simulink model "sim_demo"  (Simulink 8.2)
settings: Solver=ode45  StartTime=0.0  StopTime=10.0  RelTol=1e-3
libraries: simulink x1
settings Model: Creator=DR_C  LastModifiedBy=DR_C
settings DebuggingCC: FcnCallInpInsideContextMsg=EnableAllAsWarning
settings GRTTargetCC: CombineOutputUpdateFcns=on  GRTInterface=off

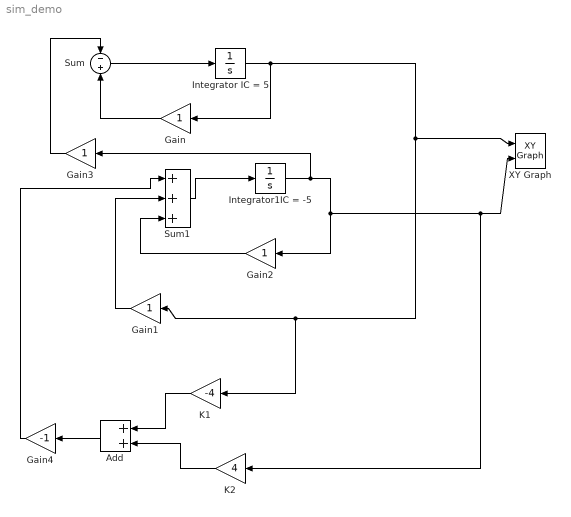
== system sim_demo ==
  Add : Sum
  Gain{,1..3} (4 alike) : Gain
  Gain4 : Gain  Gain=-1
  Integrator IC = 5 : Integrator  InitialCondition=5
  Integrator1IC = -5 : Integrator  InitialCondition=-5
  K1 : Gain  Gain=-4
  K2 : Gain  Gain=4
  Sum : Sum  Inputs=-+
  Sum1 : Sum  Inputs=+++
  XY Graph : simulink/Sinks/XY Graph  xmin=-10  xmax=10  ymin=-10  ymax=10  st=-1
  wires:
  Sum/1 -> Integrator IC = 5/1
  Gain/1 -> Sum/2
  Integrator IC = 5/1 -> Gain/1, XY Graph/1, Gain1/1, K1/1
  Sum1/1 -> Integrator1IC = -5/1
  Integrator1IC = -5/1 -> Gain3/1, Gain2/1, XY Graph/2, K2/1
  Gain3/1 -> Sum/1
  Gain2/1 -> Sum1/3
  Gain1/1 -> Sum1/2
  K1/1 -> Add/1
  K2/1 -> Add/2
  Add/1 -> Gain4/1
  Gain4/1 -> Sum1/1
